simulink model "RLC2"  (R2015a)
settings: Solver=ode4  StartTime=0.0  StopTime=10.0  FixedStep=0.0001  RelTol=1e-3
settings Model: Creator=Aranya Dan  LastModifiedBy=Aranya Dan

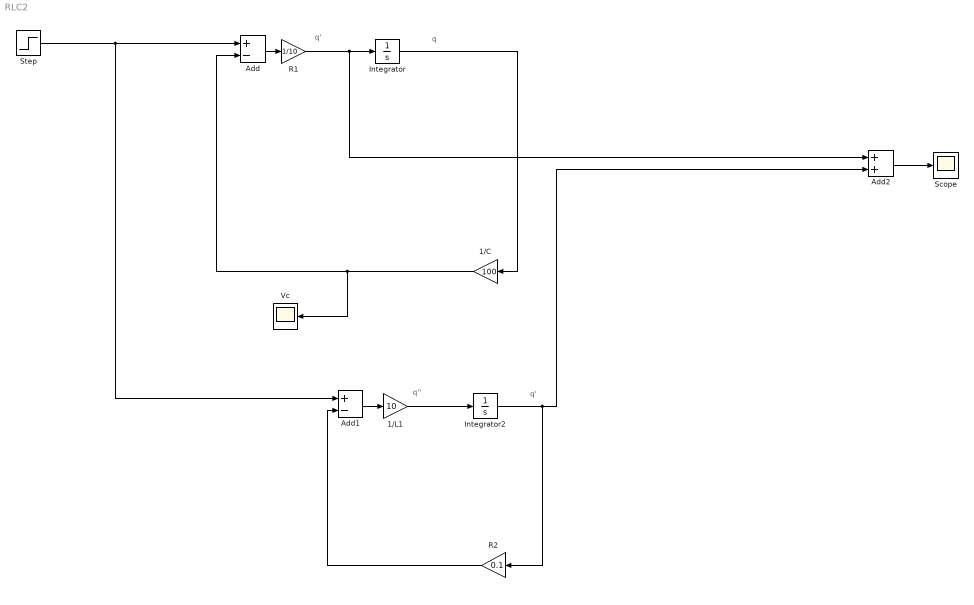
== system RLC2 ==
  note: q'
  note: q
  note: q''
  note: q'
  1/C : Gain  Gain=100
  1/L1 : Gain  Gain=10
  Add : Sum  Inputs=+-
  Add1 : Sum  Inputs=+-
  Add2 : Sum
  Integrator : Integrator
  Integrator2 : Integrator
  R1 : Gain  Gain=1/10
  R2 : Gain  Gain=0.1
  Scope : Scope
  Step : Step  Time=0  After=10  SampleTime=0
  Vc : Scope
  wires:
  Integrator/1 -> 1/C/1
  Add/1 -> R1/1
  1/C/1 -> Add/2, Vc/1
  Integrator2/1 -> R2/1, Add2/2
  Add1/1 -> 1/L1/1
  R2/1 -> Add1/2
  Step/1 -> Add1/1, Add/1
  1/L1/1 -> Integrator2/1
  Add2/1 -> Scope/1
  R1/1 -> Add2/1, Integrator/1
